simulink model "task2"  (R2022b)
settings: Solver=VariableStepAuto  StartTime=0.0  StopTime=20  RelTol=1e-3
libraries: cstblocks x6
settings Model: Creator=mrxmi  LastModifiedBy=mrxmi

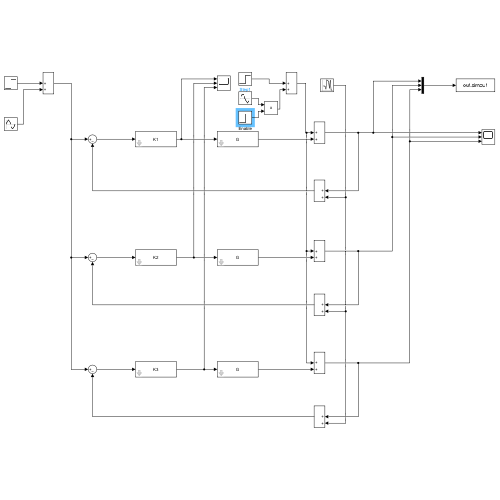
[thumbnail: Simulink's stored preview of the top-level diagram]
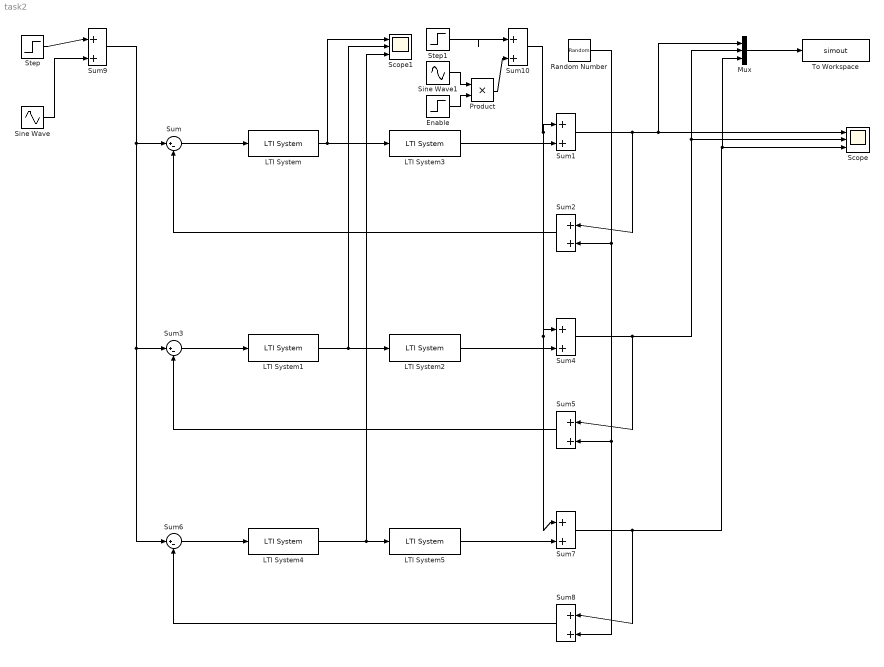
== system task2 ==
  Enable : Step  Time=10  After=0  SampleTime=0
  LTI System : cstblocks/LTI System  sys=K1  IC=[]
  LTI System1 : cstblocks/LTI System  sys=K2  IC=[]
  LTI System2 : cstblocks/LTI System  sys=G  IC=[]
  LTI System3 : cstblocks/LTI System  sys=G  IC=[]
  LTI System4 : cstblocks/LTI System  sys=K3  IC=[]
  LTI System5 : cstblocks/LTI System  sys=G  IC=[]
  Mux : Mux  Inputs=3
  Product : Product
  Random Number : RandomNumber  Variance=0  SampleTime=0.1
  Scope : Scope  NumInputPorts=3
  Scope1 : Scope  NumInputPorts=3
  Sine Wave : Sin  SampleTime=0
  Sine Wave1 : Sin  SampleTime=0
  Step : Step  Time=0  After=0  SampleTime=0
  Step1 : Step  Time=10  After=0  SampleTime=0
  Sum : Sum  Inputs=|+-
  Sum{1..2,4..5,7..10} (8 alike) : Sum  Inputs=|++
  Sum3 : Sum  Inputs=|+-
  Sum6 : Sum  Inputs=|+-
  To Workspace : ToWorkspace  VariableName=simout  SaveFormat=Structure With Time  SampleTime=-1
  wires:
  LTI System/1 -> Scope1/1, LTI System3/1
  LTI System3/1 -> Sum1/2
  Sum1/1 -> Mux/1, Scope/1, Sum2/1
  Sum2/1 -> Sum/2
  Sum/1 -> LTI System/1
  Sum3/1 -> LTI System1/1
  LTI System1/1 -> Scope1/2, LTI System2/1
  Sum4/1 -> Mux/2, Scope/2, Sum5/1
  LTI System2/1 -> Sum4/2
  Sum5/1 -> Sum3/2
  Step/1 -> Sum9/1
  Sum6/1 -> LTI System4/1
  LTI System4/1 -> Scope1/3, LTI System5/1
  Sum7/1 -> Sum8/1, Mux/3, Scope/3
  LTI System5/1 -> Sum7/2
  Sum8/1 -> Sum6/2
  Mux/1 -> To Workspace/1
  Random Number/1 -> Sum8/2, Sum5/2, Sum2/2
  Sine Wave/1 -> Sum9/2
  Sum9/1 -> Sum6/1, Sum3/1, Sum/1
  Step1/1 -> Sum10/1
  Sum10/1 -> Sum7/1, Sum4/1, Sum1/1
  Enable/1 -> Product/2
  Sine Wave1/1 -> Product/1
  Product/1 -> Sum10/2
